simulink model "adc16_dbf_4fft"  (R2013a)
settings: Solver=ode45  StartTime=0.0  StopTime=2050  RelTol=1e-3
undefined symbols (not defined in the file): pfb_coeff_gen_calc
libraries: xbsIndex_r4 x1713, casper_library_misc x294, casper_library_delays x48, casper_library_pfbs x16, simulink x16, xps_library x1
(part 3 of 21)

== system adc16_dbf_4fft/pfb_single_channel2 ==
  sync : Inport
  pol1_in : Inport  Port=2
  pol2_in : Inport  Port=3
  pol3_in : Inport  Port=4
  pol4_in : Inport  Port=5
  Terminator : Terminator
  Terminator1 : Terminator
  Terminator2 : Terminator
  pfb_fir_real1 : Subsystem  Tag=casper:pfb_fir_real  AncestorBlock=casper_library_pfbs/pfb_fir_real  mask(pfb_fir_real){PFBSize=2, TotalTaps=4, WindowType=hamming, n_inputs=0, MakeBiplex=off, BitWidthIn=8, BitWidthOut=18, CoeffBitWidth=18, CoeffDistMem=off, add_latency=1, mult_latency=2, bram_latency=2, fan_latency=1, conv_latency=1, quantization=Round  (unbiased: Even Values), fwidth=1, mult_spec=2, adder_folding=on, adder_imp=Fabric, coeffs_share=off}
      mask prompts: PFBSize "Size of PFB: (2^? pnts)"; TotalTaps "Total Number of Taps:"; WindowType "Windowing Function:"; n_inputs "Number of Simultaneous Inputs: (2^?)"; MakeBiplex "Make Biplex?"; BitWidthIn "Input Bitwidth:"; BitWidthOut "Output Bitwidth:"; CoeffBitWidth "Coefficient Bitwidth:"; CoeffDistMem "Use Distributed Memory for Coeffs"; add_latency "Add Latency"; mult_latency "Mult Latency"; bram_latency "BRAM Latency"; fan_latency "Fanout latency"; conv_latency "Convert latency"; quantization "Quantization Behavior"; fwidth "Bin Width Scaling (normal=1)"; mult_spec "Multiplier specification (0=core, 1=embedded, 2=behavioural) (left=1st tap, or just one value)"; adder_folding "Fold adders into DSPs"; adder_imp "Adder implementation"; coeffs_share "Share coefficients between polarisations (use less BRAM)?"
      mask help:
      | Fold adders into DSPs: Causes adders to be absorbed into DSP blocks (supported in Virtex5)
      | Adder implementation: Cores using Fabric or DSP48 or behavioral HDL
      mask init: same as adc16_dbf_4fft/pfb_single_channel/pfb_fir_real1
      settings: AttributesFormatString=taps=4, add_latency=1
      mask Help: eval('xlWeb(''http://casper.berkeley.edu/wiki/Pfb_fir_real'')')
      mask Callback TotalTaps:
      | %num_taps = eval(get_param(gcb, 'TotalTaps'));
      | %old_vec = eval(get_param(gcb, 'mult_spec'));=-0l
      | 
      | %vec = 2.*ones(1,num_taps);
      | %old_size = length(old_vec);
      | 
      | %if(old_size <= num_taps),
      | %    new_size = old_size;
      | %else,
      | %    new_size = num_taps;
      | %end
      | 
      | %for n = 1:new_size, vec(n) = old_vec(n); end
      | %set_param(gcb, 'mult_spec', mat2str(vec));
      mask TypeOptions WindowType: bartlett | barthannwin | blackman | blackmanharris | bohamwin | chebwin | flattopwin | gausswin | hamming | hann | kaiser | nuttallwin | parzenwin | rectwin | tukeywin | triang | userwindow
      mask TypeOptions quantization: Truncate | Round  (unbiased: +/- Inf) | Round  (unbiased: Even Values)
      mask TypeOptions adder_imp: Behavioral | Fabric | DSP48
  pfb_fir_real2 : Subsystem  Tag=casper:pfb_fir_real  AncestorBlock=casper_library_pfbs/pfb_fir_real  mask(pfb_fir_real){PFBSize=2, TotalTaps=4, WindowType=hamming, n_inputs=0, MakeBiplex=off, BitWidthIn=8, BitWidthOut=18, CoeffBitWidth=18, CoeffDistMem=off, add_latency=1, mult_latency=2, bram_latency=2, fan_latency=1, conv_latency=1, quantization=Round  (unbiased: Even Values), fwidth=1, mult_spec=2, adder_folding=on, adder_imp=Fabric, coeffs_share=off}
      mask prompts: PFBSize "Size of PFB: (2^? pnts)"; TotalTaps "Total Number of Taps:"; WindowType "Windowing Function:"; n_inputs "Number of Simultaneous Inputs: (2^?)"; MakeBiplex "Make Biplex?"; BitWidthIn "Input Bitwidth:"; BitWidthOut "Output Bitwidth:"; CoeffBitWidth "Coefficient Bitwidth:"; CoeffDistMem "Use Distributed Memory for Coeffs"; add_latency "Add Latency"; mult_latency "Mult Latency"; bram_latency "BRAM Latency"; fan_latency "Fanout latency"; conv_latency "Convert latency"; quantization "Quantization Behavior"; fwidth "Bin Width Scaling (normal=1)"; mult_spec "Multiplier specification (0=core, 1=embedded, 2=behavioural) (left=1st tap, or just one value)"; adder_folding "Fold adders into DSPs"; adder_imp "Adder implementation"; coeffs_share "Share coefficients between polarisations (use less BRAM)?"
      mask help:
      | Fold adders into DSPs: Causes adders to be absorbed into DSP blocks (supported in Virtex5)
      | Adder implementation: Cores using Fabric or DSP48 or behavioral HDL
      mask init: same as adc16_dbf_4fft/pfb_single_channel/pfb_fir_real1
      settings: AttributesFormatString=taps=4, add_latency=1
      mask Help: eval('xlWeb(''http://casper.berkeley.edu/wiki/Pfb_fir_real'')')
      mask Callback TotalTaps:
      | %num_taps = eval(get_param(gcb, 'TotalTaps'));
      | %old_vec = eval(get_param(gcb, 'mult_spec'));=-0l
      | 
      | %vec = 2.*ones(1,num_taps);
      | %old_size = length(old_vec);
      | 
      | %if(old_size <= num_taps),
      | %    new_size = old_size;
      | %else,
      | %    new_size = num_taps;
      | %end
      | 
      | %for n = 1:new_size, vec(n) = old_vec(n); end
      | %set_param(gcb, 'mult_spec', mat2str(vec));
      mask TypeOptions WindowType: bartlett | barthannwin | blackman | blackmanharris | bohamwin | chebwin | flattopwin | gausswin | hamming | hann | kaiser | nuttallwin | parzenwin | rectwin | tukeywin | triang | userwindow
      mask TypeOptions quantization: Truncate | Round  (unbiased: +/- Inf) | Round  (unbiased: Even Values)
      mask TypeOptions adder_imp: Behavioral | Fabric | DSP48
  pfb_fir_real3 : Subsystem  Tag=casper:pfb_fir_real  AncestorBlock=casper_library_pfbs/pfb_fir_real  mask(pfb_fir_real){PFBSize=2, TotalTaps=4, WindowType=hamming, n_inputs=0, MakeBiplex=off, BitWidthIn=8, BitWidthOut=18, CoeffBitWidth=18, CoeffDistMem=off, add_latency=1, mult_latency=2, bram_latency=2, fan_latency=1, conv_latency=1, quantization=Round  (unbiased: Even Values), fwidth=1, mult_spec=2, adder_folding=on, adder_imp=Fabric, coeffs_share=off}
      mask prompts: PFBSize "Size of PFB: (2^? pnts)"; TotalTaps "Total Number of Taps:"; WindowType "Windowing Function:"; n_inputs "Number of Simultaneous Inputs: (2^?)"; MakeBiplex "Make Biplex?"; BitWidthIn "Input Bitwidth:"; BitWidthOut "Output Bitwidth:"; CoeffBitWidth "Coefficient Bitwidth:"; CoeffDistMem "Use Distributed Memory for Coeffs"; add_latency "Add Latency"; mult_latency "Mult Latency"; bram_latency "BRAM Latency"; fan_latency "Fanout latency"; conv_latency "Convert latency"; quantization "Quantization Behavior"; fwidth "Bin Width Scaling (normal=1)"; mult_spec "Multiplier specification (0=core, 1=embedded, 2=behavioural) (left=1st tap, or just one value)"; adder_folding "Fold adders into DSPs"; adder_imp "Adder implementation"; coeffs_share "Share coefficients between polarisations (use less BRAM)?"
      mask help:
      | Fold adders into DSPs: Causes adders to be absorbed into DSP blocks (supported in Virtex5)
      | Adder implementation: Cores using Fabric or DSP48 or behavioral HDL
      mask init: same as adc16_dbf_4fft/pfb_single_channel/pfb_fir_real1
      settings: AttributesFormatString=taps=4, add_latency=1
      mask Help: eval('xlWeb(''http://casper.berkeley.edu/wiki/Pfb_fir_real'')')
      mask Callback TotalTaps:
      | %num_taps = eval(get_param(gcb, 'TotalTaps'));
      | %old_vec = eval(get_param(gcb, 'mult_spec'));=-0l
      | 
      | %vec = 2.*ones(1,num_taps);
      | %old_size = length(old_vec);
      | 
      | %if(old_size <= num_taps),
      | %    new_size = old_size;
      | %else,
      | %    new_size = num_taps;
      | %end
      | 
      | %for n = 1:new_size, vec(n) = old_vec(n); end
      | %set_param(gcb, 'mult_spec', mat2str(vec));
      mask TypeOptions WindowType: bartlett | barthannwin | blackman | blackmanharris | bohamwin | chebwin | flattopwin | gausswin | hamming | hann | kaiser | nuttallwin | parzenwin | rectwin | tukeywin | triang | userwindow
      mask TypeOptions quantization: Truncate | Round  (unbiased: +/- Inf) | Round  (unbiased: Even Values)
      mask TypeOptions adder_imp: Behavioral | Fabric | DSP48
  pfb_fir_real4 : Subsystem  Tag=casper:pfb_fir_real  AncestorBlock=casper_library_pfbs/pfb_fir_real  mask(pfb_fir_real){PFBSize=2, TotalTaps=4, WindowType=hamming, n_inputs=0, MakeBiplex=off, BitWidthIn=8, BitWidthOut=18, CoeffBitWidth=18, CoeffDistMem=off, add_latency=1, mult_latency=2, bram_latency=2, fan_latency=1, conv_latency=1, quantization=Round  (unbiased: Even Values), fwidth=1, mult_spec=2, adder_folding=on, adder_imp=Fabric, coeffs_share=off}
      mask prompts: PFBSize "Size of PFB: (2^? pnts)"; TotalTaps "Total Number of Taps:"; WindowType "Windowing Function:"; n_inputs "Number of Simultaneous Inputs: (2^?)"; MakeBiplex "Make Biplex?"; BitWidthIn "Input Bitwidth:"; BitWidthOut "Output Bitwidth:"; CoeffBitWidth "Coefficient Bitwidth:"; CoeffDistMem "Use Distributed Memory for Coeffs"; add_latency "Add Latency"; mult_latency "Mult Latency"; bram_latency "BRAM Latency"; fan_latency "Fanout latency"; conv_latency "Convert latency"; quantization "Quantization Behavior"; fwidth "Bin Width Scaling (normal=1)"; mult_spec "Multiplier specification (0=core, 1=embedded, 2=behavioural) (left=1st tap, or just one value)"; adder_folding "Fold adders into DSPs"; adder_imp "Adder implementation"; coeffs_share "Share coefficients between polarisations (use less BRAM)?"
      mask help:
      | Fold adders into DSPs: Causes adders to be absorbed into DSP blocks (supported in Virtex5)
      | Adder implementation: Cores using Fabric or DSP48 or behavioral HDL
      mask init: same as adc16_dbf_4fft/pfb_single_channel/pfb_fir_real1
      settings: AttributesFormatString=taps=4, add_latency=1
      mask Help: eval('xlWeb(''http://casper.berkeley.edu/wiki/Pfb_fir_real'')')
      mask Callback TotalTaps:
      | %num_taps = eval(get_param(gcb, 'TotalTaps'));
      | %old_vec = eval(get_param(gcb, 'mult_spec'));=-0l
      | 
      | %vec = 2.*ones(1,num_taps);
      | %old_size = length(old_vec);
      | 
      | %if(old_size <= num_taps),
      | %    new_size = old_size;
      | %else,
      | %    new_size = num_taps;
      | %end
      | 
      | %for n = 1:new_size, vec(n) = old_vec(n); end
      | %set_param(gcb, 'mult_spec', mat2str(vec));
      mask TypeOptions WindowType: bartlett | barthannwin | blackman | blackmanharris | bohamwin | chebwin | flattopwin | gausswin | hamming | hann | kaiser | nuttallwin | parzenwin | rectwin | tukeywin | triang | userwindow
      mask TypeOptions quantization: Truncate | Round  (unbiased: +/- Inf) | Round  (unbiased: Even Values)
      mask TypeOptions adder_imp: Behavioral | Fabric | DSP48
  sync_out : Outport
  pol1_out : Outport  Port=2
  pol2_out : Outport  Port=3
  pol3_out : Outport  Port=4
  pol4_out : Outport  Port=5
  wires:
  pol2_in/1 -> pfb_fir_real2/2(pol1_in1)
  pol3_in/1 -> pfb_fir_real3/2(pol1_in1)
  pfb_fir_real1/2(pol1_out1) -> pol1_out/1
  sync/1 -> pfb_fir_real4/1(sync), pfb_fir_real3/1(sync), pfb_fir_real2/1(sync), pfb_fir_real1/1(sync)
  pfb_fir_real3/2(pol1_out1) -> pol3_out/1
  pfb_fir_real4/2(pol1_out1) -> pol4_out/1
  pol1_in/1 -> pfb_fir_real1/2(pol1_in1)
  pol4_in/1 -> pfb_fir_real4/2(pol1_in1)
  pfb_fir_real2/2(pol1_out1) -> pol2_out/1
  pfb_fir_real1/1(sync_out) -> sync_out/1
  pfb_fir_real2/1(sync_out) -> Terminator/1
  pfb_fir_real3/1(sync_out) -> Terminator1/1
  pfb_fir_real4/1(sync_out) -> Terminator2/1

== system adc16_dbf_4fft/pfb_single_channel3 ==
  sync : Inport
  pol1_in : Inport  Port=2
  pol2_in : Inport  Port=3
  pol3_in : Inport  Port=4
  pol4_in : Inport  Port=5
  Terminator : Terminator
  Terminator1 : Terminator
  Terminator2 : Terminator
  pfb_fir_real1 : Subsystem  Tag=casper:pfb_fir_real  AncestorBlock=casper_library_pfbs/pfb_fir_real  mask(pfb_fir_real){PFBSize=2, TotalTaps=4, WindowType=hamming, n_inputs=0, MakeBiplex=off, BitWidthIn=8, BitWidthOut=18, CoeffBitWidth=18, CoeffDistMem=off, add_latency=1, mult_latency=2, bram_latency=2, fan_latency=1, conv_latency=1, quantization=Round  (unbiased: Even Values), fwidth=1, mult_spec=2, adder_folding=on, adder_imp=Fabric, coeffs_share=off}
      mask prompts: PFBSize "Size of PFB: (2^? pnts)"; TotalTaps "Total Number of Taps:"; WindowType "Windowing Function:"; n_inputs "Number of Simultaneous Inputs: (2^?)"; MakeBiplex "Make Biplex?"; BitWidthIn "Input Bitwidth:"; BitWidthOut "Output Bitwidth:"; CoeffBitWidth "Coefficient Bitwidth:"; CoeffDistMem "Use Distributed Memory for Coeffs"; add_latency "Add Latency"; mult_latency "Mult Latency"; bram_latency "BRAM Latency"; fan_latency "Fanout latency"; conv_latency "Convert latency"; quantization "Quantization Behavior"; fwidth "Bin Width Scaling (normal=1)"; mult_spec "Multiplier specification (0=core, 1=embedded, 2=behavioural) (left=1st tap, or just one value)"; adder_folding "Fold adders into DSPs"; adder_imp "Adder implementation"; coeffs_share "Share coefficients between polarisations (use less BRAM)?"
      mask help:
      | Fold adders into DSPs: Causes adders to be absorbed into DSP blocks (supported in Virtex5)
      | Adder implementation: Cores using Fabric or DSP48 or behavioral HDL
      mask init: same as adc16_dbf_4fft/pfb_single_channel/pfb_fir_real1
      settings: AttributesFormatString=taps=4, add_latency=1
      mask Help: eval('xlWeb(''http://casper.berkeley.edu/wiki/Pfb_fir_real'')')
      mask Callback TotalTaps:
      | %num_taps = eval(get_param(gcb, 'TotalTaps'));
      | %old_vec = eval(get_param(gcb, 'mult_spec'));=-0l
      | 
      | %vec = 2.*ones(1,num_taps);
      | %old_size = length(old_vec);
      | 
      | %if(old_size <= num_taps),
      | %    new_size = old_size;
      | %else,
      | %    new_size = num_taps;
      | %end
      | 
      | %for n = 1:new_size, vec(n) = old_vec(n); end
      | %set_param(gcb, 'mult_spec', mat2str(vec));
      mask TypeOptions WindowType: bartlett | barthannwin | blackman | blackmanharris | bohamwin | chebwin | flattopwin | gausswin | hamming | hann | kaiser | nuttallwin | parzenwin | rectwin | tukeywin | triang | userwindow
      mask TypeOptions quantization: Truncate | Round  (unbiased: +/- Inf) | Round  (unbiased: Even Values)
      mask TypeOptions adder_imp: Behavioral | Fabric | DSP48
  pfb_fir_real2 : Subsystem  Tag=casper:pfb_fir_real  AncestorBlock=casper_library_pfbs/pfb_fir_real  mask(pfb_fir_real){PFBSize=2, TotalTaps=4, WindowType=hamming, n_inputs=0, MakeBiplex=off, BitWidthIn=8, BitWidthOut=18, CoeffBitWidth=18, CoeffDistMem=off, add_latency=1, mult_latency=2, bram_latency=2, fan_latency=1, conv_latency=1, quantization=Round  (unbiased: Even Values), fwidth=1, mult_spec=2, adder_folding=on, adder_imp=Fabric, coeffs_share=off}
      mask prompts: PFBSize "Size of PFB: (2^? pnts)"; TotalTaps "Total Number of Taps:"; WindowType "Windowing Function:"; n_inputs "Number of Simultaneous Inputs: (2^?)"; MakeBiplex "Make Biplex?"; BitWidthIn "Input Bitwidth:"; BitWidthOut "Output Bitwidth:"; CoeffBitWidth "Coefficient Bitwidth:"; CoeffDistMem "Use Distributed Memory for Coeffs"; add_latency "Add Latency"; mult_latency "Mult Latency"; bram_latency "BRAM Latency"; fan_latency "Fanout latency"; conv_latency "Convert latency"; quantization "Quantization Behavior"; fwidth "Bin Width Scaling (normal=1)"; mult_spec "Multiplier specification (0=core, 1=embedded, 2=behavioural) (left=1st tap, or just one value)"; adder_folding "Fold adders into DSPs"; adder_imp "Adder implementation"; coeffs_share "Share coefficients between polarisations (use less BRAM)?"
      mask help:
      | Fold adders into DSPs: Causes adders to be absorbed into DSP blocks (supported in Virtex5)
      | Adder implementation: Cores using Fabric or DSP48 or behavioral HDL
      mask init: same as adc16_dbf_4fft/pfb_single_channel/pfb_fir_real1
      settings: AttributesFormatString=taps=4, add_latency=1
      mask Help: eval('xlWeb(''http://casper.berkeley.edu/wiki/Pfb_fir_real'')')
      mask Callback TotalTaps:
      | %num_taps = eval(get_param(gcb, 'TotalTaps'));
      | %old_vec = eval(get_param(gcb, 'mult_spec'));=-0l
      | 
      | %vec = 2.*ones(1,num_taps);
      | %old_size = length(old_vec);
      | 
      | %if(old_size <= num_taps),
      | %    new_size = old_size;
      | %else,
      | %    new_size = num_taps;
      | %end
      | 
      | %for n = 1:new_size, vec(n) = old_vec(n); end
      | %set_param(gcb, 'mult_spec', mat2str(vec));
      mask TypeOptions WindowType: bartlett | barthannwin | blackman | blackmanharris | bohamwin | chebwin | flattopwin | gausswin | hamming | hann | kaiser | nuttallwin | parzenwin | rectwin | tukeywin | triang | userwindow
      mask TypeOptions quantization: Truncate | Round  (unbiased: +/- Inf) | Round  (unbiased: Even Values)
      mask TypeOptions adder_imp: Behavioral | Fabric | DSP48
  pfb_fir_real3 : Subsystem  Tag=casper:pfb_fir_real  AncestorBlock=casper_library_pfbs/pfb_fir_real  mask(pfb_fir_real){PFBSize=2, TotalTaps=4, WindowType=hamming, n_inputs=0, MakeBiplex=off, BitWidthIn=8, BitWidthOut=18, CoeffBitWidth=18, CoeffDistMem=off, add_latency=1, mult_latency=2, bram_latency=2, fan_latency=1, conv_latency=1, quantization=Round  (unbiased: Even Values), fwidth=1, mult_spec=2, adder_folding=on, adder_imp=Fabric, coeffs_share=off}
      mask prompts: PFBSize "Size of PFB: (2^? pnts)"; TotalTaps "Total Number of Taps:"; WindowType "Windowing Function:"; n_inputs "Number of Simultaneous Inputs: (2^?)"; MakeBiplex "Make Biplex?"; BitWidthIn "Input Bitwidth:"; BitWidthOut "Output Bitwidth:"; CoeffBitWidth "Coefficient Bitwidth:"; CoeffDistMem "Use Distributed Memory for Coeffs"; add_latency "Add Latency"; mult_latency "Mult Latency"; bram_latency "BRAM Latency"; fan_latency "Fanout latency"; conv_latency "Convert latency"; quantization "Quantization Behavior"; fwidth "Bin Width Scaling (normal=1)"; mult_spec "Multiplier specification (0=core, 1=embedded, 2=behavioural) (left=1st tap, or just one value)"; adder_folding "Fold adders into DSPs"; adder_imp "Adder implementation"; coeffs_share "Share coefficients between polarisations (use less BRAM)?"
      mask help:
      | Fold adders into DSPs: Causes adders to be absorbed into DSP blocks (supported in Virtex5)
      | Adder implementation: Cores using Fabric or DSP48 or behavioral HDL
      mask init: same as adc16_dbf_4fft/pfb_single_channel/pfb_fir_real1
      settings: AttributesFormatString=taps=4, add_latency=1
      mask Help: eval('xlWeb(''http://casper.berkeley.edu/wiki/Pfb_fir_real'')')
      mask Callback TotalTaps:
      | %num_taps = eval(get_param(gcb, 'TotalTaps'));
      | %old_vec = eval(get_param(gcb, 'mult_spec'));=-0l
      | 
      | %vec = 2.*ones(1,num_taps);
      | %old_size = length(old_vec);
      | 
      | %if(old_size <= num_taps),
      | %    new_size = old_size;
      | %else,
      | %    new_size = num_taps;
      | %end
      | 
      | %for n = 1:new_size, vec(n) = old_vec(n); end
      | %set_param(gcb, 'mult_spec', mat2str(vec));
      mask TypeOptions WindowType: bartlett | barthannwin | blackman | blackmanharris | bohamwin | chebwin | flattopwin | gausswin | hamming | hann | kaiser | nuttallwin | parzenwin | rectwin | tukeywin | triang | userwindow
      mask TypeOptions quantization: Truncate | Round  (unbiased: +/- Inf) | Round  (unbiased: Even Values)
      mask TypeOptions adder_imp: Behavioral | Fabric | DSP48
  pfb_fir_real4 : Subsystem  Tag=casper:pfb_fir_real  AncestorBlock=casper_library_pfbs/pfb_fir_real  mask(pfb_fir_real){PFBSize=2, TotalTaps=4, WindowType=hamming, n_inputs=0, MakeBiplex=off, BitWidthIn=8, BitWidthOut=18, CoeffBitWidth=18, CoeffDistMem=off, add_latency=1, mult_latency=2, bram_latency=2, fan_latency=1, conv_latency=1, quantization=Round  (unbiased: Even Values), fwidth=1, mult_spec=2, adder_folding=on, adder_imp=Fabric, coeffs_share=off}
      mask prompts: PFBSize "Size of PFB: (2^? pnts)"; TotalTaps "Total Number of Taps:"; WindowType "Windowing Function:"; n_inputs "Number of Simultaneous Inputs: (2^?)"; MakeBiplex "Make Biplex?"; BitWidthIn "Input Bitwidth:"; BitWidthOut "Output Bitwidth:"; CoeffBitWidth "Coefficient Bitwidth:"; CoeffDistMem "Use Distributed Memory for Coeffs"; add_latency "Add Latency"; mult_latency "Mult Latency"; bram_latency "BRAM Latency"; fan_latency "Fanout latency"; conv_latency "Convert latency"; quantization "Quantization Behavior"; fwidth "Bin Width Scaling (normal=1)"; mult_spec "Multiplier specification (0=core, 1=embedded, 2=behavioural) (left=1st tap, or just one value)"; adder_folding "Fold adders into DSPs"; adder_imp "Adder implementation"; coeffs_share "Share coefficients between polarisations (use less BRAM)?"
      mask help:
      | Fold adders into DSPs: Causes adders to be absorbed into DSP blocks (supported in Virtex5)
      | Adder implementation: Cores using Fabric or DSP48 or behavioral HDL
      mask init: same as adc16_dbf_4fft/pfb_single_channel/pfb_fir_real1
      settings: AttributesFormatString=taps=4, add_latency=1
      mask Help: eval('xlWeb(''http://casper.berkeley.edu/wiki/Pfb_fir_real'')')
      mask Callback TotalTaps:
      | %num_taps = eval(get_param(gcb, 'TotalTaps'));
      | %old_vec = eval(get_param(gcb, 'mult_spec'));=-0l
      | 
      | %vec = 2.*ones(1,num_taps);
      | %old_size = length(old_vec);
      | 
      | %if(old_size <= num_taps),
      | %    new_size = old_size;
      | %else,
      | %    new_size = num_taps;
      | %end
      | 
      | %for n = 1:new_size, vec(n) = old_vec(n); end
      | %set_param(gcb, 'mult_spec', mat2str(vec));
      mask TypeOptions WindowType: bartlett | barthannwin | blackman | blackmanharris | bohamwin | chebwin | flattopwin | gausswin | hamming | hann | kaiser | nuttallwin | parzenwin | rectwin | tukeywin | triang | userwindow
      mask TypeOptions quantization: Truncate | Round  (unbiased: +/- Inf) | Round  (unbiased: Even Values)
      mask TypeOptions adder_imp: Behavioral | Fabric | DSP48
  sync_out : Outport
  pol1_out : Outport  Port=2
  pol2_out : Outport  Port=3
  pol3_out : Outport  Port=4
  pol4_out : Outport  Port=5
  wires:
  pfb_fir_real4/1(sync_out) -> Terminator2/1
  pfb_fir_real3/1(sync_out) -> Terminator1/1
  pfb_fir_real2/1(sync_out) -> Terminator/1
  pfb_fir_real1/1(sync_out) -> sync_out/1
  pfb_fir_real2/2(pol1_out1) -> pol2_out/1
  pol4_in/1 -> pfb_fir_real4/2(pol1_in1)
  pol1_in/1 -> pfb_fir_real1/2(pol1_in1)
  pfb_fir_real4/2(pol1_out1) -> pol4_out/1
  pfb_fir_real3/2(pol1_out1) -> pol3_out/1
  sync/1 -> pfb_fir_real1/1(sync), pfb_fir_real2/1(sync), pfb_fir_real3/1(sync), pfb_fir_real4/1(sync)
  pfb_fir_real1/2(pol1_out1) -> pol1_out/1
  pol3_in/1 -> pfb_fir_real3/2(pol1_in1)
  pol2_in/1 -> pfb_fir_real2/2(pol1_in1)

== system adc16_dbf_4fft/power2scope ==
  In1 : Inport
  In2 : Inport  Port=2
  In3 : Inport  Port=3
  In4 : Inport  Port=4
  Bus Creator16 : BusCreator
  gateway17 : Subsystem
  power{,1..3} (4 alike) : casper_library_misc/power  BitWidth=18  add_latency=2  mult_latency=3
  Out1 : Outport
  wires:
  gateway17/1(to_scope) -> Out1/1
  power2/1 -> Bus Creator16/3
  In3/1 -> power2/1
  In4/1 -> power3/1
  Bus Creator16/1 -> gateway17/1(data[4])
  In2/1 -> power1/1
  power1/1 -> Bus Creator16/2
  power3/1 -> Bus Creator16/4
  power/1 -> Bus Creator16/1
  In1/1 -> power/1

== system adc16_dbf_4fft/power2scope1 ==
  In1 : Inport
  In2 : Inport  Port=2
  In3 : Inport  Port=3
  In4 : Inport  Port=4
  Bus Creator16 : BusCreator
  gateway17 : Subsystem
  power{,1..3} (4 alike) : casper_library_misc/power  BitWidth=18  add_latency=2  mult_latency=3
  Out1 : Outport
  wires:
  In1/1 -> power/1
  power/1 -> Bus Creator16/1
  power3/1 -> Bus Creator16/4
  power1/1 -> Bus Creator16/2
  In2/1 -> power1/1
  Bus Creator16/1 -> gateway17/1(data[4])
  In4/1 -> power3/1
  In3/1 -> power2/1
  power2/1 -> Bus Creator16/3
  gateway17/1(to_scope) -> Out1/1

== system adc16_dbf_4fft/power2scope2 ==
  In1 : Inport
  In2 : Inport  Port=2
  In3 : Inport  Port=3
  In4 : Inport  Port=4
  Bus Creator16 : BusCreator
  gateway17 : Subsystem
  power{,1..3} (4 alike) : casper_library_misc/power  BitWidth=18  add_latency=2  mult_latency=3
  Out1 : Outport
  wires:
  gateway17/1(to_scope) -> Out1/1
  power2/1 -> Bus Creator16/3
  In3/1 -> power2/1
  In4/1 -> power3/1
  Bus Creator16/1 -> gateway17/1(data[4])
  In2/1 -> power1/1
  power1/1 -> Bus Creator16/2
  power3/1 -> Bus Creator16/4
  power/1 -> Bus Creator16/1
  In1/1 -> power/1

== system adc16_dbf_4fft/power2scope3 ==
  In1 : Inport
  In2 : Inport  Port=2
  In3 : Inport  Port=3
  In4 : Inport  Port=4
  Bus Creator16 : BusCreator
  gateway17 : Subsystem
  power{,1..3} (4 alike) : casper_library_misc/power  BitWidth=18  add_latency=2  mult_latency=3
  Out1 : Outport
  wires:
  In1/1 -> power/1
  power/1 -> Bus Creator16/1
  power3/1 -> Bus Creator16/4
  power1/1 -> Bus Creator16/2
  In2/1 -> power1/1
  Bus Creator16/1 -> gateway17/1(data[4])
  In4/1 -> power3/1
  In3/1 -> power2/1
  power2/1 -> Bus Creator16/3
  gateway17/1(to_scope) -> Out1/1

== system adc16_dbf_4fft/power2scope4 ==
  In1 : Inport
  In2 : Inport  Port=2
  In3 : Inport  Port=3
  In4 : Inport  Port=4
  Bus Creator16 : BusCreator
  gateway17 : Subsystem
  power{,1..3} (4 alike) : casper_library_misc/power  BitWidth=18  add_latency=2  mult_latency=3
  Out1 : Outport
  wires:
  In1/1 -> power/1
  power/1 -> Bus Creator16/1
  power3/1 -> Bus Creator16/4
  power1/1 -> Bus Creator16/2
  In2/1 -> power1/1
  Bus Creator16/1 -> gateway17/1(data[4])
  In4/1 -> power3/1
  In3/1 -> power2/1
  power2/1 -> Bus Creator16/3
  gateway17/1(to_scope) -> Out1/1

== system adc16_dbf_4fft/power2scope5 ==
  In1 : Inport
  In2 : Inport  Port=2
  In3 : Inport  Port=3
  In4 : Inport  Port=4
  Bus Creator16 : BusCreator
  gateway17 : Subsystem
  power{,1..3} (4 alike) : casper_library_misc/power  BitWidth=18  add_latency=2  mult_latency=3
  Out1 : Outport
  wires:
  gateway17/1(to_scope) -> Out1/1
  power2/1 -> Bus Creator16/3
  In3/1 -> power2/1
  In4/1 -> power3/1
  Bus Creator16/1 -> gateway17/1(data[4])
  In2/1 -> power1/1
  power1/1 -> Bus Creator16/2
  power3/1 -> Bus Creator16/4
  power/1 -> Bus Creator16/1
  In1/1 -> power/1

== system adc16_dbf_4fft/power2scope6 ==
  In1 : Inport
  In2 : Inport  Port=2
  In3 : Inport  Port=3
  In4 : Inport  Port=4
  Bus Creator16 : BusCreator
  gateway17 : Subsystem
  power{,1..3} (4 alike) : casper_library_misc/power  BitWidth=18  add_latency=2  mult_latency=3
  Out1 : Outport
  wires:
  In1/1 -> power/1
  power/1 -> Bus Creator16/1
  power3/1 -> Bus Creator16/4
  power1/1 -> Bus Creator16/2
  In2/1 -> power1/1
  Bus Creator16/1 -> gateway17/1(data[4])
  In4/1 -> power3/1
  In3/1 -> power2/1
  power2/1 -> Bus Creator16/3
  gateway17/1(to_scope) -> Out1/1

== system adc16_dbf_4fft/power2scope7 ==
  In1 : Inport
  In2 : Inport  Port=2
  In3 : Inport  Port=3
  In4 : Inport  Port=4
  Bus Creator16 : BusCreator
  gateway17 : Subsystem
  power{,1..3} (4 alike) : casper_library_misc/power  BitWidth=18  add_latency=2  mult_latency=3
  Out1 : Outport
  wires:
  gateway17/1(to_scope) -> Out1/1
  power2/1 -> Bus Creator16/3
  In3/1 -> power2/1
  In4/1 -> power3/1
  Bus Creator16/1 -> gateway17/1(data[4])
  In2/1 -> power1/1
  power1/1 -> Bus Creator16/2
  power3/1 -> Bus Creator16/4
  power/1 -> Bus Creator16/1
  In1/1 -> power/1

== system adc16_dbf_4fft/power_integrator_16x ==
  chan_a : Inport
  chan_b : Inport  Port=2
  chan_c : Inport  Port=3
  chan_d : Inport  Port=4
  acc_len : Inport  Port=5
  Bus Creator{,1..3} (4 alike) : BusCreator
  Bus Selector : BusSelector  OutputSignals=a1,a2,a3,a4
  Bus Selector1 : BusSelector  OutputSignals=b1,b2,b3,b4
  Bus Selector2 : BusSelector  OutputSignals=c1,c2,c3,c4
  Bus Selector3 : BusSelector  OutputSignals=d1,d2,d3,d4
  Terminator : Terminator
  Terminator1 : Terminator
  Terminator2 : Terminator
  power_integrator_4x : Subsystem
  power_integrator_4x1 : Subsystem
  power_integrator_4x2 : Subsystem
  power_integrator_4x3 : Subsystem
  rst_out : Outport
  power_a : Outport  Port=2
  power_b : Outport  Port=3
  power_c : Outport  Port=4
  power_d : Outport  Port=5
  wires:
  power_integrator_4x/1(rst) -> rst_out/1
  acc_len/1 -> power_integrator_4x3/5(acc_len), power_integrator_4x2/5(acc_len), power_integrator_4x1/5(acc_len), power_integrator_4x/5(acc_len)
  Bus Selector/4 -> power_integrator_4x/4(in4)  "<a4>"
  Bus Selector/2 -> power_integrator_4x/2(in2)  "<a2>"
  Bus Selector/3 -> power_integrator_4x/3(in3)  "<a3>"
  Bus Selector/1 -> power_integrator_4x/1(in1)  "<a1>"
  chan_a/1 -> Bus Selector/1
  Bus Selector1/4 -> power_integrator_4x1/4(in4)  "<b4>"
  Bus Selector1/1 -> power_integrator_4x1/1(in1)  "<b1>"
  Bus Selector1/3 -> power_integrator_4x1/3(in3)  "<b3>"
  Bus Selector1/2 -> power_integrator_4x1/2(in2)  "<b2>"
  chan_b/1 -> Bus Selector1/1
  chan_d/1 -> Bus Selector3/1
  chan_c/1 -> Bus Selector2/1
  Bus Selector2/2 -> power_integrator_4x2/2(in2)  "<c2>"
  Bus Selector2/3 -> power_integrator_4x2/3(in3)  "<c3>"
  Bus Selector2/1 -> power_integrator_4x2/1(in1)  "<c1>"
  Bus Selector2/4 -> power_integrator_4x2/4(in4)  "<c4>"
  Bus Selector3/3 -> power_integrator_4x3/3(in3)  "<d3>"
  Bus Selector3/1 -> power_integrator_4x3/1(in1)  "<d1>"
  Bus Selector3/2 -> power_integrator_4x3/2(in2)  "<d2>"
  Bus Selector3/4 -> power_integrator_4x3/4(in4)  "<d4>"
  power_integrator_4x1/1(rst) -> Terminator/1
  power_integrator_4x2/1(rst) -> Terminator1/1
  power_integrator_4x3/1(rst) -> Terminator2/1
  power_integrator_4x/3(pow2) -> Bus Creator/2
  power_integrator_4x/5(pow4) -> Bus Creator/4
  power_integrator_4x/4(pow3) -> Bus Creator/3
  power_integrator_4x/2(pow1) -> Bus Creator/1
  Bus Creator/1 -> power_a/1
  power_integrator_4x1/3(pow2) -> Bus Creator1/2
  power_integrator_4x1/2(pow1) -> Bus Creator1/1
  power_integrator_4x1/5(pow4) -> Bus Creator1/4
  power_integrator_4x1/4(pow3) -> Bus Creator1/3
  Bus Creator1/1 -> power_b/1
  power_integrator_4x2/5(pow4) -> Bus Creator2/4
  power_integrator_4x2/4(pow3) -> Bus Creator2/3
  power_integrator_4x2/3(pow2) -> Bus Creator2/2
  power_integrator_4x2/2(pow1) -> Bus Creator2/1
  Bus Creator2/1 -> power_c/1
  power_integrator_4x3/5(pow4) -> Bus Creator3/4
  power_integrator_4x3/2(pow1) -> Bus Creator3/1
  power_integrator_4x3/4(pow3) -> Bus Creator3/3
  power_integrator_4x3/3(pow2) -> Bus Creator3/2
  Bus Creator3/1 -> power_d/1

== system adc16_dbf_4fft/power_integrator_4x ==
  in1 : Inport
  in2 : Inport  Port=2
  in3 : Inport  Port=3
  in4 : Inport  Port=4
  acc_len : Inport  Port=5
  Terminator : Terminator
  Terminator1 : Terminator
  Terminator2 : Terminator
  power_integrator : Subsystem
  power_integrator1 : Subsystem
  power_integrator2 : Subsystem
  power_integrator3 : Subsystem
  rst : Outport
  pow1 : Outport  Port=2
  pow2 : Outport  Port=3
  pow3 : Outport  Port=4
  pow4 : Outport  Port=5
  wires:
  power_integrator1/2(rst_out) -> Terminator/1
  power_integrator2/2(rst_out) -> Terminator1/1
  power_integrator3/2(rst_out) -> Terminator2/1
  power_integrator/1(pow) -> pow1/1
  in1/1 -> power_integrator/1(signal)
  in2/1 -> power_integrator1/1(signal)
  in3/1 -> power_integrator2/1(signal)
  in4/1 -> power_integrator3/1(signal)
  power_integrator3/1(pow) -> pow4/1
  power_integrator2/1(pow) -> pow3/1
  power_integrator1/1(pow) -> pow2/1
  power_integrator/2(rst_out) -> rst/1
  acc_len/1 -> power_integrator3/2(acc_len), power_integrator2/2(acc_len), power_integrator1/2(acc_len), power_integrator/2(acc_len)

== system adc16_dbf_4fft/power_integrator_4x1 ==
  in1 : Inport
  in2 : Inport  Port=2
  in3 : Inport  Port=3
  in4 : Inport  Port=4
  acc_len : Inport  Port=5
  Terminator : Terminator
  Terminator1 : Terminator
  Terminator2 : Terminator
  power_integrator : Subsystem
  power_integrator1 : Subsystem
  power_integrator2 : Subsystem
  power_integrator3 : Subsystem
  rst : Outport
  pow1 : Outport  Port=2
  pow2 : Outport  Port=3
  pow3 : Outport  Port=4
  pow4 : Outport  Port=5
  wires:
  acc_len/1 -> power_integrator/2(acc_len), power_integrator1/2(acc_len), power_integrator2/2(acc_len), power_integrator3/2(acc_len)
  power_integrator/2(rst_out) -> rst/1
  power_integrator1/1(pow) -> pow2/1
  power_integrator2/1(pow) -> pow3/1
  power_integrator3/1(pow) -> pow4/1
  in4/1 -> power_integrator3/1(signal)
  in3/1 -> power_integrator2/1(signal)
  in2/1 -> power_integrator1/1(signal)
  in1/1 -> power_integrator/1(signal)
  power_integrator/1(pow) -> pow1/1
  power_integrator3/2(rst_out) -> Terminator2/1
  power_integrator2/2(rst_out) -> Terminator1/1
  power_integrator1/2(rst_out) -> Terminator/1

== system adc16_dbf_4fft/power_integrator_4x2 ==
  in1 : Inport
  in2 : Inport  Port=2
  in3 : Inport  Port=3
  in4 : Inport  Port=4
  acc_len : Inport  Port=5
  Terminator : Terminator
  Terminator1 : Terminator
  Terminator2 : Terminator
  power_integrator : Subsystem
  power_integrator1 : Subsystem
  power_integrator2 : Subsystem
  power_integrator3 : Subsystem
  rst : Outport
  pow1 : Outport  Port=2
  pow2 : Outport  Port=3
  pow3 : Outport  Port=4
  pow4 : Outport  Port=5
  wires:
  power_integrator1/2(rst_out) -> Terminator/1
  power_integrator2/2(rst_out) -> Terminator1/1
  power_integrator3/2(rst_out) -> Terminator2/1
  power_integrator/1(pow) -> pow1/1
  in1/1 -> power_integrator/1(signal)
  in2/1 -> power_integrator1/1(signal)
  in3/1 -> power_integrator2/1(signal)
  in4/1 -> power_integrator3/1(signal)
  power_integrator3/1(pow) -> pow4/1
  power_integrator2/1(pow) -> pow3/1
  power_integrator1/1(pow) -> pow2/1
  power_integrator/2(rst_out) -> rst/1
  acc_len/1 -> power_integrator3/2(acc_len), power_integrator2/2(acc_len), power_integrator1/2(acc_len), power_integrator/2(acc_len)

== system adc16_dbf_4fft/power_integrator_4x3 ==
  in1 : Inport
  in2 : Inport  Port=2
  in3 : Inport  Port=3
  in4 : Inport  Port=4
  acc_len : Inport  Port=5
  Terminator : Terminator
  Terminator1 : Terminator
  Terminator2 : Terminator
  power_integrator : Subsystem
  power_integrator1 : Subsystem
  power_integrator2 : Subsystem
  power_integrator3 : Subsystem
  rst : Outport
  pow1 : Outport  Port=2
  pow2 : Outport  Port=3
  pow3 : Outport  Port=4
  pow4 : Outport  Port=5
  wires:
  acc_len/1 -> power_integrator/2(acc_len), power_integrator1/2(acc_len), power_integrator2/2(acc_len), power_integrator3/2(acc_len)
  power_integrator/2(rst_out) -> rst/1
  power_integrator1/1(pow) -> pow2/1
  power_integrator2/1(pow) -> pow3/1
  power_integrator3/1(pow) -> pow4/1
  in4/1 -> power_integrator3/1(signal)
  in3/1 -> power_integrator2/1(signal)
  in2/1 -> power_integrator1/1(signal)
  in1/1 -> power_integrator/1(signal)
  power_integrator/1(pow) -> pow1/1
  power_integrator3/2(rst_out) -> Terminator2/1
  power_integrator2/2(rst_out) -> Terminator1/1
  power_integrator1/2(rst_out) -> Terminator/1

== system adc16_dbf_4fft/sine_with_noise1 ==
  Add : Sum
  Band-Limited White Noise : simulink/Sources/Band-Limited White Noise  Cov=[0.001]  Ts=1  seed=[232]
  Sine Wave : Sin  SineType=Sample based  Samples=25  SampleTime=1
  Out1 : Outport
  wires:
  Sine Wave/1 -> Add/1
  Add/1 -> Out1/1
  Band-Limited White Noise/1 -> Add/2

== system adc16_dbf_4fft/sine_with_noise10 ==
  Add : Sum
  Band-Limited White Noise : simulink/Sources/Band-Limited White Noise  Cov=[0.001]  Ts=1  seed=[232]
  Sine Wave : Sin  SineType=Sample based  Samples=25  SampleTime=1
  Out1 : Outport
  wires:
  Sine Wave/1 -> Add/1
  Add/1 -> Out1/1
  Band-Limited White Noise/1 -> Add/2

== system adc16_dbf_4fft/sine_with_noise11 ==
  Add : Sum
  Band-Limited White Noise : simulink/Sources/Band-Limited White Noise  Cov=[0.001]  Ts=1  seed=[232]
  Sine Wave : Sin  SineType=Sample based  Samples=25  SampleTime=1
  Out1 : Outport
  wires:
  Band-Limited White Noise/1 -> Add/2
  Add/1 -> Out1/1
  Sine Wave/1 -> Add/1

== system adc16_dbf_4fft/sine_with_noise12 ==
  Add : Sum
  Band-Limited White Noise : simulink/Sources/Band-Limited White Noise  Cov=[0.001]  Ts=1  seed=[232]
  Sine Wave : Sin  SineType=Sample based  Samples=25  SampleTime=1
  Out1 : Outport
  wires:
  Sine Wave/1 -> Add/1
  Add/1 -> Out1/1
  Band-Limited White Noise/1 -> Add/2

== system adc16_dbf_4fft/sine_with_noise13 ==
  Add : Sum
  Band-Limited White Noise : simulink/Sources/Band-Limited White Noise  Cov=[0.001]  Ts=1  seed=[232]
  Sine Wave : Sin  SineType=Sample based  Samples=25  SampleTime=1
  Out1 : Outport
  wires:
  Band-Limited White Noise/1 -> Add/2
  Add/1 -> Out1/1
  Sine Wave/1 -> Add/1

== system adc16_dbf_4fft/sine_with_noise14 ==
  Add : Sum
  Band-Limited White Noise : simulink/Sources/Band-Limited White Noise  Cov=[0.001]  Ts=1  seed=[232]
  Sine Wave : Sin  SineType=Sample based  Samples=25  SampleTime=1
  Out1 : Outport
  wires:
  Band-Limited White Noise/1 -> Add/2
  Add/1 -> Out1/1
  Sine Wave/1 -> Add/1

== system adc16_dbf_4fft/sine_with_noise15 ==
  Add : Sum
  Band-Limited White Noise : simulink/Sources/Band-Limited White Noise  Cov=[0.001]  Ts=1  seed=[232]
  Sine Wave : Sin  SineType=Sample based  Samples=25  SampleTime=1
  Out1 : Outport
  wires:
  Sine Wave/1 -> Add/1
  Add/1 -> Out1/1
  Band-Limited White Noise/1 -> Add/2

== system adc16_dbf_4fft/sine_with_noise17 ==
  Add : Sum
  Band-Limited White Noise : simulink/Sources/Band-Limited White Noise  Cov=[0.001]  Ts=1  seed=[232]
  Sine Wave : Sin  SineType=Sample based  Samples=25  SampleTime=1
  Out1 : Outport
  wires:
  Band-Limited White Noise/1 -> Add/2
  Add/1 -> Out1/1
  Sine Wave/1 -> Add/1

== system adc16_dbf_4fft/sine_with_noise2 ==
  Add : Sum
  Band-Limited White Noise : simulink/Sources/Band-Limited White Noise  Cov=[0.001]  Ts=1  seed=[232]
  Sine Wave : Sin  SineType=Sample based  Samples=25  SampleTime=1
  Out1 : Outport
  wires:
  Band-Limited White Noise/1 -> Add/2
  Add/1 -> Out1/1
  Sine Wave/1 -> Add/1

== system adc16_dbf_4fft/sine_with_noise3 ==
  Add : Sum
  Band-Limited White Noise : simulink/Sources/Band-Limited White Noise  Cov=[0.001]  Ts=1  seed=[232]
  Sine Wave : Sin  SineType=Sample based  Samples=25  SampleTime=1
  Out1 : Outport
  wires:
  Sine Wave/1 -> Add/1
  Add/1 -> Out1/1
  Band-Limited White Noise/1 -> Add/2

== system adc16_dbf_4fft/sine_with_noise4 ==
  Add : Sum
  Band-Limited White Noise : simulink/Sources/Band-Limited White Noise  Cov=[0.001]  Ts=1  seed=[232]
  Sine Wave : Sin  SineType=Sample based  Samples=25  SampleTime=1
  Out1 : Outport
  wires:
  Band-Limited White Noise/1 -> Add/2
  Add/1 -> Out1/1
  Sine Wave/1 -> Add/1

== system adc16_dbf_4fft/sine_with_noise5 ==
  Add : Sum
  Band-Limited White Noise : simulink/Sources/Band-Limited White Noise  Cov=[0.001]  Ts=1  seed=[232]
  Sine Wave : Sin  SineType=Sample based  Samples=25  SampleTime=1
  Out1 : Outport
  wires:
  Sine Wave/1 -> Add/1
  Add/1 -> Out1/1
  Band-Limited White Noise/1 -> Add/2

== system adc16_dbf_4fft/sine_with_noise6 ==
  Add : Sum
  Band-Limited White Noise : simulink/Sources/Band-Limited White Noise  Cov=[0.001]  Ts=1  seed=[232]
  Sine Wave : Sin  SineType=Sample based  Samples=25  SampleTime=1
  Out1 : Outport
  wires:
  Sine Wave/1 -> Add/1
  Add/1 -> Out1/1
  Band-Limited White Noise/1 -> Add/2

== system adc16_dbf_4fft/sine_with_noise7 ==
  Add : Sum
  Band-Limited White Noise : simulink/Sources/Band-Limited White Noise  Cov=[0.001]  Ts=1  seed=[232]
  Sine Wave : Sin  SineType=Sample based  Samples=25  SampleTime=1
  Out1 : Outport
  wires:
  Band-Limited White Noise/1 -> Add/2
  Add/1 -> Out1/1
  Sine Wave/1 -> Add/1

== system adc16_dbf_4fft/sine_with_noise8 ==
  Add : Sum
  Band-Limited White Noise : simulink/Sources/Band-Limited White Noise  Cov=[0.001]  Ts=1  seed=[232]
  Sine Wave : Sin  SineType=Sample based  Samples=25  SampleTime=1
  Out1 : Outport
  wires:
  Band-Limited White Noise/1 -> Add/2
  Add/1 -> Out1/1
  Sine Wave/1 -> Add/1

== system adc16_dbf_4fft/sine_with_noise9 ==
  Add : Sum
  Band-Limited White Noise : simulink/Sources/Band-Limited White Noise  Cov=[0.001]  Ts=1  seed=[232]
  Sine Wave : Sin  SineType=Sample based  Samples=25  SampleTime=1
  Out1 : Outport
  wires:
  Sine Wave/1 -> Add/1
  Add/1 -> Out1/1
  Band-Limited White Noise/1 -> Add/2

== system adc16_dbf_4fft/snap ==
  data_a : Inport
  data_b : Inport  Port=2
  data_c : Inport  Port=3
  data_d : Inport  Port=4
  trig : Inport  Port=5
  Bus Selector : BusSelector  OutputSignals=a1,a2,a3,a4
  Bus Selector1 : BusSelector  OutputSignals=b1,b2,b3,b4
  Bus Selector2 : BusSelector  OutputSignals=c1,c2,c3,c4
  Bus Selector3 : BusSelector  OutputSignals=d1,d2,d3,d4
  Constant : xbsIndex_r4/Constant  const=0  gui_display_data_type=Boolean  arith_type=Boolean  n_bits=16  bin_pt=14  preci_type=Single  exp_width=8  frac_width=24  explicit_period=off  period=1  equ=P=C  opselect=C  inp2=PCIN>>17  opr=+  inp1=P  carry=CIN  dbl_ovrd=off  block_type=constant
  a : Subsystem  Tag=casper:snapshot  AncestorBlock=casper_library_scopes/snapshot  mask(snapshot){storage=bram, dram_dimm=1, dram_clock=200, nsamples=16, data_width=32, offset=off, circap=off, value=off, use_dsp48=on}
      mask prompts: storage "Storage medium"; dram_dimm "DRAM dimm"; dram_clock "DRAM clock rate"; nsamples "Number of Samples (2^?)"; data_width "Data width"; offset "Start delay support"; circap "Circular capture support"; value "Extra value capture support"; use_dsp48 "Use DSP48s to implement counters"
      mask help:
      | Standard snap block, but with the following optional extras;
      |  1) Optionally delay the fabric trigger by a user-specified number of valids.
      |  2) Capture continuously after a trigger until a stop pulse is received. Data is captured into BRAM continuously, with old data being overwritten until a stop command is received. Then stop capturing when memory is filled. This enables you to get some data before and some data after the stop pulse. Use the 'tr_en_cnt' register to determine where you are in your vector. 'Addr' register's MSb now indicates 'busy capturing'.
      |  3) Optionally capture a value on an input port to a register at the same time as the first data sample.
      |  4) Implement counters using DSP48Es to save resources.
      mask init:
      | snapshot_init(gcb, ...
      |     'storage', storage, ...
      |     'dram_dimm', dram_dimm, ...
      |     'dram_clock', dram_clock, ...
      |     'nsamples', nsamples, ...
      |     'data_width', data_width, ...
      |     'offset', offset, ...
      |     'circap', circap, ...
      |     'value', value, ...
      |     'use_dsp48', use_dsp48);
      mask TypeOptions storage: bram | dram
      mask Callback storage: snapshot_callback();
      mask TypeOptions dram_dimm: 1 | 2 | 3 | 4
      mask TypeOptions dram_clock: 200 | 250 | 266 | 300 | 333
      mask TypeOptions data_width: 8 | 16 | 32 | 64 | 128
  b : Subsystem  Tag=casper:snapshot  AncestorBlock=casper_library_scopes/snapshot  mask(snapshot){storage=bram, dram_dimm=1, dram_clock=200, nsamples=16, data_width=32, offset=off, circap=off, value=off, use_dsp48=on}
      mask prompts: storage "Storage medium"; dram_dimm "DRAM dimm"; dram_clock "DRAM clock rate"; nsamples "Number of Samples (2^?)"; data_width "Data width"; offset "Start delay support"; circap "Circular capture support"; value "Extra value capture support"; use_dsp48 "Use DSP48s to implement counters"
      mask help:
      | Standard snap block, but with the following optional extras;
      |  1) Optionally delay the fabric trigger by a user-specified number of valids.
      |  2) Capture continuously after a trigger until a stop pulse is received. Data is captured into BRAM continuously, with old data being overwritten until a stop command is received. Then stop capturing when memory is filled. This enables you to get some data before and some data after the stop pulse. Use the 'tr_en_cnt' register to determine where you are in your vector. 'Addr' register's MSb now indicates 'busy capturing'.
      |  3) Optionally capture a value on an input port to a register at the same time as the first data sample.
      |  4) Implement counters using DSP48Es to save resources.
      mask init: same as adc16_dbf_4fft/snap/a
      mask TypeOptions storage: bram | dram
      mask Callback storage: snapshot_callback();
      mask TypeOptions dram_dimm: 1 | 2 | 3 | 4
      mask TypeOptions dram_clock: 200 | 250 | 266 | 300 | 333
      mask TypeOptions data_width: 8 | 16 | 32 | 64 | 128
  bus_create : Subsystem  AncestorBlock=casper_library_flow_control/bus_create  mask(bus_create){inputNum=4}
      mask prompts: inputNum "Number of inputs:"
      mask init:
      | bus_create_init(gcb,...
      |     'inputNum', inputNum);
  bus_create1 : Subsystem  AncestorBlock=casper_library_flow_control/bus_create  mask(bus_create){inputNum=4}
      mask prompts: inputNum "Number of inputs:"
      mask init:
      | bus_create_init(gcb,...
      |     'inputNum', inputNum);
  bus_create2 : Subsystem  AncestorBlock=casper_library_flow_control/bus_create  mask(bus_create){inputNum=4}
      mask prompts: inputNum "Number of inputs:"
      mask init:
      | bus_create_init(gcb,...
      |     'inputNum', inputNum);
  bus_create3 : Subsystem  AncestorBlock=casper_library_flow_control/bus_create  mask(bus_create){inputNum=4}
      mask prompts: inputNum "Number of inputs:"
      mask init:
      | bus_create_init(gcb,...
      |     'inputNum', inputNum);
  c : Subsystem  Tag=casper:snapshot  AncestorBlock=casper_library_scopes/snapshot  mask(snapshot){storage=bram, dram_dimm=1, dram_clock=200, nsamples=16, data_width=32, offset=off, circap=off, value=off, use_dsp48=on}
      mask prompts: storage "Storage medium"; dram_dimm "DRAM dimm"; dram_clock "DRAM clock rate"; nsamples "Number of Samples (2^?)"; data_width "Data width"; offset "Start delay support"; circap "Circular capture support"; value "Extra value capture support"; use_dsp48 "Use DSP48s to implement counters"
      mask help:
      | Standard snap block, but with the following optional extras;
      |  1) Optionally delay the fabric trigger by a user-specified number of valids.
      |  2) Capture continuously after a trigger until a stop pulse is received. Data is captured into BRAM continuously, with old data being overwritten until a stop command is received. Then stop capturing when memory is filled. This enables you to get some data before and some data after the stop pulse. Use the 'tr_en_cnt' register to determine where you are in your vector. 'Addr' register's MSb now indicates 'busy capturing'.
      |  3) Optionally capture a value on an input port to a register at the same time as the first data sample.
      |  4) Implement counters using DSP48Es to save resources.
      mask init: same as adc16_dbf_4fft/snap/a
      mask TypeOptions storage: bram | dram
      mask Callback storage: snapshot_callback();
      mask TypeOptions dram_dimm: 1 | 2 | 3 | 4
      mask TypeOptions dram_clock: 200 | 250 | 266 | 300 | 333
      mask TypeOptions data_width: 8 | 16 | 32 | 64 | 128
  d : Subsystem  Tag=casper:snapshot  AncestorBlock=casper_library_scopes/snapshot  mask(snapshot){storage=bram, dram_dimm=1, dram_clock=200, nsamples=16, data_width=32, offset=off, circap=off, value=off, use_dsp48=on}
      mask prompts: storage "Storage medium"; dram_dimm "DRAM dimm"; dram_clock "DRAM clock rate"; nsamples "Number of Samples (2^?)"; data_width "Data width"; offset "Start delay support"; circap "Circular capture support"; value "Extra value capture support"; use_dsp48 "Use DSP48s to implement counters"
      mask help:
      | Standard snap block, but with the following optional extras;
      |  1) Optionally delay the fabric trigger by a user-specified number of valids.
      |  2) Capture continuously after a trigger until a stop pulse is received. Data is captured into BRAM continuously, with old data being overwritten until a stop command is received. Then stop capturing when memory is filled. This enables you to get some data before and some data after the stop pulse. Use the 'tr_en_cnt' register to determine where you are in your vector. 'Addr' register's MSb now indicates 'busy capturing'.
      |  3) Optionally capture a value on an input port to a register at the same time as the first data sample.
      |  4) Implement counters using DSP48Es to save resources.
      mask init: same as adc16_dbf_4fft/snap/a
      mask TypeOptions storage: bram | dram
      mask Callback storage: snapshot_callback();
      mask TypeOptions dram_dimm: 1 | 2 | 3 | 4
      mask TypeOptions dram_clock: 200 | 250 | 266 | 300 | 333
      mask TypeOptions data_width: 8 | 16 | 32 | 64 | 128
  wires:
  Constant/1 -> d/2(we), c/2(we), b/2(we), a/2(we)
  trig/1 -> a/3(trig), b/3(trig), c/3(trig), d/3(trig)
  Bus Selector/3 -> bus_create/3(in3)  "<a3>"
  Bus Selector/1 -> bus_create/1(in1)  "<a1>"
  Bus Selector/2 -> bus_create/2(in2)  "<a2>"
  Bus Selector/4 -> bus_create/4(in4)  "<a4>"
  bus_create/1(bus_out) -> a/1(din)
  Bus Selector1/3 -> bus_create1/3(in3)  "<b3>"
  Bus Selector1/4 -> bus_create1/4(in4)  "<b4>"
  Bus Selector1/1 -> bus_create1/1(in1)  "<b1>"
  Bus Selector1/2 -> bus_create1/2(in2)  "<b2>"
  Bus Selector2/1 -> bus_create2/1(in1)  "<c1>"
  Bus Selector2/2 -> bus_create2/2(in2)  "<c2>"
  Bus Selector2/3 -> bus_create2/3(in3)  "<c3>"
  Bus Selector2/4 -> bus_create2/4(in4)  "<c4>"
  Bus Selector3/1 -> bus_create3/1(in1)  "<d1>"
  Bus Selector3/2 -> bus_create3/2(in2)  "<d2>"
  Bus Selector3/3 -> bus_create3/3(in3)  "<d3>"
  Bus Selector3/4 -> bus_create3/4(in4)  "<d4>"
  bus_create3/1(bus_out) -> d/1(din)
  bus_create2/1(bus_out) -> c/1(din)
  bus_create1/1(bus_out) -> b/1(din)
  data_a/1 -> Bus Selector/1
  data_d/1 -> Bus Selector3/1
  data_c/1 -> Bus Selector2/1
  data_b/1 -> Bus Selector1/1
